simulink model "uno1"  (R2012b)
settings: Solver=ode45  StartTime=0.0  StopTime=20.0  RelTol=1e-3
settings Model: Creator=Daniel  LastModifiedBy=Daniel

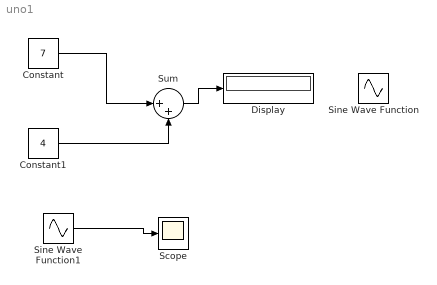
== system uno1 ==
  Constant : Constant  Value=7
  Constant1 : Constant  Value=4
  Display : Display
  Scope : Scope
      settings: TimeRange=10  YMin=-9
  Sine Wave Function : Sin  TimeSource=Use external signal  SampleTime=0
  Sine Wave Function1 : Sin  Amplitude=2  Frequency=30  SampleTime=.1
  Sum : Sum  Inputs=|++
  wires:
  Constant/1 -> Sum/1
  Constant1/1 -> Sum/2
  Sum/1 -> Display/1
  Sine Wave Function1/1 -> Scope/1
